simulink library "satAttKinematics_sl"  (R2023b)
settings: Solver=VariableStepAuto  StartTime=0.0  StopTime=10.0  RelTol=1e-3
libraries: vrlib x1
settings Model: Creator=gilbu  LastModifiedBy=gilbu

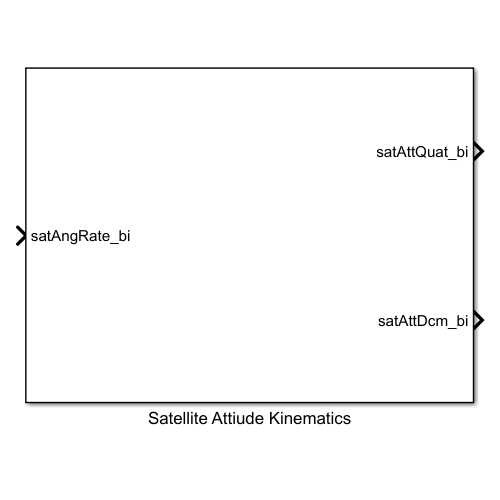
[thumbnail: Simulink's stored preview of the top-level diagram]
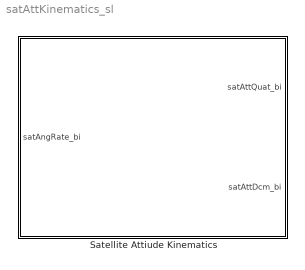
== system satAttKinematics_sl ==
  Satellite Attiude Kinematics : Subsystem  mask{satAttQuat0=0, satAttDcm0=0}
      mask prompts: satAttQuat0 "Initial Satellite Attiude Quaternion /vec scalar/"; satAttDcm0 "Inital Satellite Attitude DCM [3,3]"
      mask DialogControl DescTextVar Prompt: Satellite Attitude Kinematics Propagation. Uses DCM kinematics and quaternion kinematics. Input satelllite angular rate of body w.r.t inertial frame expressed in body cord. Outputs new attiude DCM and quaternion.

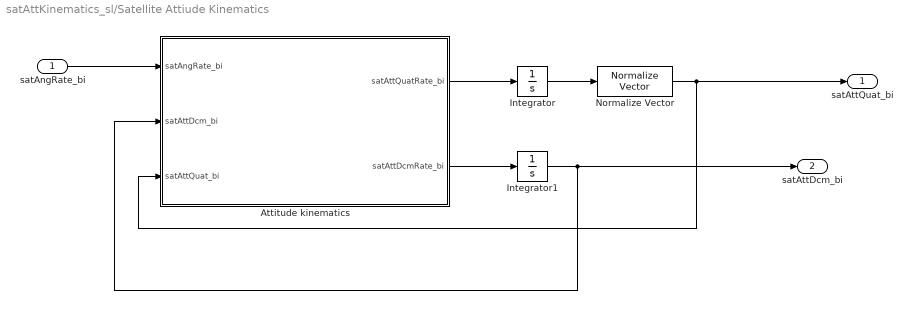
== system satAttKinematics_sl/Satellite Attiude Kinematics ==
  satAngRate_bi : Inport
  Attitude kinematics : MATLAB Function  TreatAsAtomicUnit=on
  Integrator : Integrator  InitialCondition=satAttQuat0
  Integrator1 : Integrator  InitialCondition=satAttDcm0
  Normalize Vector : vrlib/Utilities/Normalize Vector  maxzero=0
  satAttQuat_bi : Outport
  satAttDcm_bi : Outport  Port=2
  wires:
  Integrator1/1 -> satAttDcm_bi/1, Attitude kinematics/2(satAttDcm_bi)
  Attitude kinematics/1(satAttQuatRate_bi) -> Integrator/1
  Integrator/1 -> Normalize Vector/1
  Normalize Vector/1 -> satAttQuat_bi/1, Attitude kinematics/3(satAttQuat_bi)
  satAngRate_bi/1 -> Attitude kinematics/1(satAngRate_bi)
  Attitude kinematics/2(satAttDcmRate_bi) -> Integrator1/1

== matlab function satAttKinematics_sl/Satellite Attiude Kinematics/Attitude kinematics ==
  data: satAngRate_bi input size=3; satAttQuatRate_bi output size=4; satAttDcm_bi input; satAttQuat_bi input size=4; satAttDcmRate_bi output size=3,3
%satAttKinematics    Sat attitude kinematics calculations for Att, Prop
function [satAttQuatRate_bi,satAttDcmRate_bi]= satAttKinematics( ...
    satAngRate_bi,satAttDcm_bi,satAttQuat_bi ... % Inputs
    )% Parameters
%-------------------------------------------------------------------------------
% DCM Rates

% Construct angular rate skew symmetric matrix
omegaSkew = [0 -satAngRate_bi(3) satAngRate_bi(2);
             satAngRate_bi(3) 0 -satAngRate_bi(1);
             -satAngRate_bi(2) satAngRate_bi(1) 0 ];

% Calcualte DCM Rate of Change Matrix
satAttDcmRate_bi = -omegaSkew*satAttDcm_bi;

%-------------------------------------------------------------------------------
% Attitude Quaternion Rates

% Pure angular rate queaternion
satAngRateQuat_bi = [satAngRate_bi' 0]';

% Quaternion multiplication ang rate quaternion to att quaternion
satAttQuatRate_bi = 0.5*quatMult(satAngRateQuat_bi,satAttQuat_bi);

%[0 -satAngRate_bi'; satAngRate_bi -omegaSkew]*satAttQuat_bi;

end

%-------------------------------------------------------------------------------
% Auxiliary Functions

% Quaternion Multiplication
function quatProduct = quatMult(quat1,quat2)
    
    quatVec = quat2(4).*quat1(1:3)+quat1(4).*quat2(1:3) - cross(quat1(1:3),quat2(1:3));
    quatScalar = quat1(4)*quat2(4)-dot(quat1(1:3),quat2(1:3));

    quatProduct = [quatVec' quatScalar]';
end
